simulink model "Robust_design_step_validation_real"  (R2025b)
settings: Solver=ode5  StartTime=0.0  StopTime=20  FixedStep=0.001  RelTol=1e-3
undefined symbols (not defined in the file): degs2rpm, index, K_vec, National_Instruments, Nu, Nx, PCI, rdp, rpm2rads, sens, u_bar_max
libraries: sldrtlib x3
settings Model: SimulationMode=external  ExtModeTrigDuration=20001  Creator=fasoloandr  LastModifiedBy=Enrico
settings DataIOCC: ReturnWorkspaceOutputs=off
settings HardwareCC: ProdBitPerLong=64.0  ProdHWDeviceType=Intel->x86-64 (Linux 64)
settings RTWCC: SystemTargetFile=sldrt.tlc  TemplateMakefile=sldrt.tmf  RTWCompilerOptimization=on  Description=Simulink Desktop Real-Time
settings CodeAppCC: MaxIdLength=95.0
settings SimulinkDesktopRealTimeCC: ExtModeTransport=0.0  ExtModeStaticAllocSize=1000000.0  TargetLibSuffix=_sldrt.a  TargetPreCompLibLocation=D:\Programmi (D)\MATLAB\R2025b\toolbox\sldrt\lib\win64  MultiwordLength=2048.0  DynamicStringBufferSize=256.0  ParMdlRefBuildCompliant=on  PreserveMATLABNamespacesInGeneratedCode=on  SubcomponentCodeInterfacePackaging=Reusable function

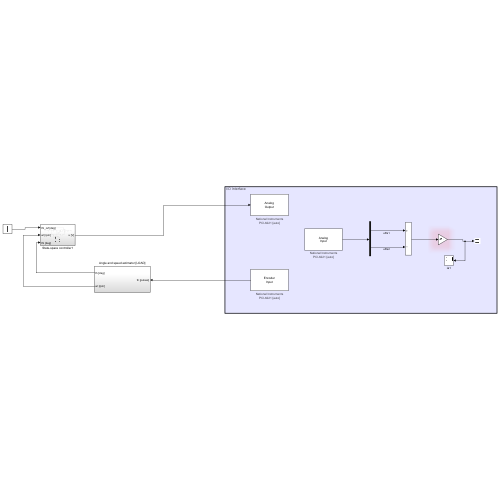
[thumbnail: Simulink's stored preview of the top-level diagram]
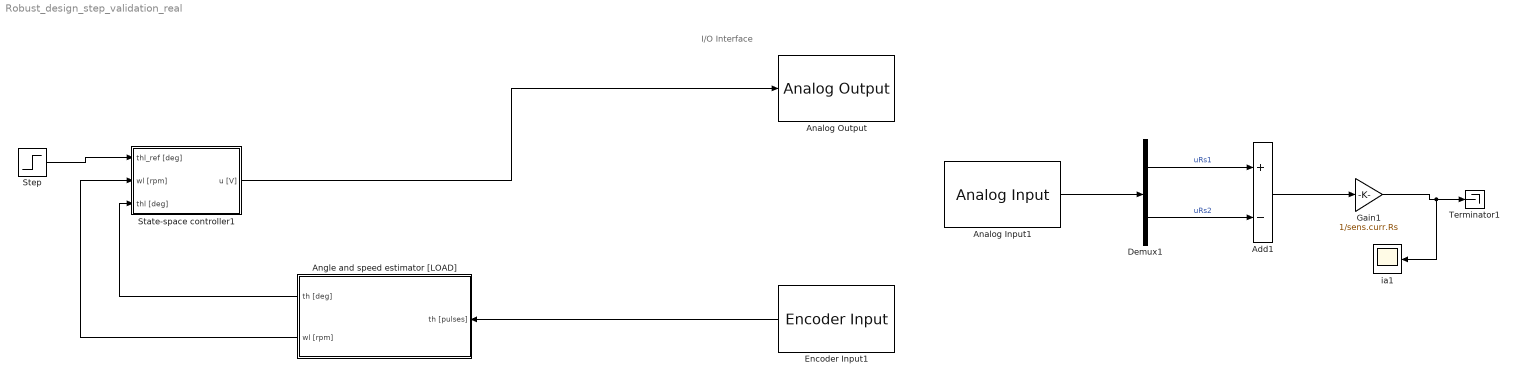
== system Robust_design_step_validation_real ==
  note: I/O Interface
  Add1 : Sum  Inputs=+-
  Analog Input1 : sldrtlib/Analog Input  SampleTime=-1  MaxMissedTicks=10  ShowMissedTicks=off  YieldWhenWaiting=off  DrvName=National_Instruments/PCI-6221  DrvAddress=4294967295  DrvOptions=[0 0 0 2 0]  Channels=[1,2]  RangeMode=1  VoltRange=1  DataType=1
      settings: AttributesFormatString=National Instruments\nPCI-6221 [auto]
  Analog Output : sldrtlib/Analog Output  SampleTime=-1  MaxMissedTicks=10  ShowMissedTicks=off  YieldWhenWaiting=off  DrvName=National_Instruments/PCI-6221  DrvAddress=4294967295  DrvOptions=[0 0 0 2 0]  Channels=1  RangeMode=1  VoltRange=1  InitialValue=[0]  FinalValue=[0]
      settings: AttributesFormatString=National Instruments\nPCI-6221 [auto]
  Angle and speed estimator [LOAD] : Subsystem
  Demux1 : Demux  Outputs=2
  Encoder Input1 : sldrtlib/Encoder Input  SampleTime=-1  MaxMissedTicks=10  ShowMissedTicks=off  YieldWhenWaiting=off  DrvName=National_Instruments/PCI-6221  DrvAddress=4294967295  DrvOptions=[0 0 0 2 0]  Channels=1  QuadMode=3  IndexPulse=1  InputFilter=Inf  DataType=1
      settings: AttributesFormatString=National Instruments\nPCI-6221 [auto]
  Gain1 : Gain  Gain=1/sens.curr.Rs
  State-space controller1 : Subsystem
  Step : Step  SampleTime=0
  Terminator1 : Terminator
  ia1 : Scope
      settings: ActiveDisplayYMinimum=-1  ActiveDisplayYMaximum=1  DataLoggingVariableName=ScopeData2
  wires:
  Add1/1 -> Gain1/1
  Demux1/1 -> Add1/1  "uRs1"
  Demux1/2 -> Add1/2  "uRs2"
  Gain1/1 -> ia1/1, Terminator1/1
  Analog Input1/1 -> Demux1/1
  Step/1 -> State-space controller1/1(thl_ref [deg])
  Angle and speed estimator [LOAD]/1(th [deg]) -> State-space controller1/3(thl [deg])
  Encoder Input1/1 -> Angle and speed estimator [LOAD]/1(th [pulses])
  Angle and speed estimator [LOAD]/2(wl [rpm]) -> State-space controller1/2(wl [rpm])
  State-space controller1/1(u [V]) -> Analog Output/1

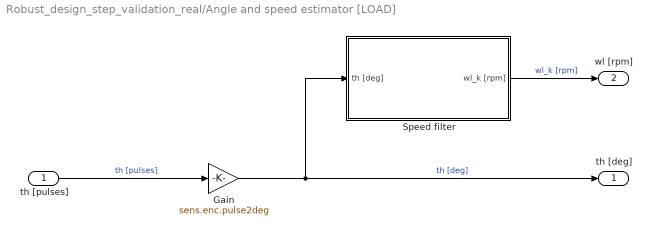
== system Robust_design_step_validation_real/Angle and speed estimator [LOAD] ==
  th [pulses] : Inport
  Gain : Gain  Gain=sens.enc.pulse2deg
  Speed filter : Subsystem
  th [deg] : Outport
  wl [rpm] : Outport  Port=2
  wires:
  Speed filter/1(wl_k [rpm]) -> wl [rpm]/1  "wl_k [rpm]"
  th [pulses]/1 -> Gain/1  "th [pulses]"
  Gain/1 -> Speed filter/1(th [deg]), th [deg]/1  "th [deg]"

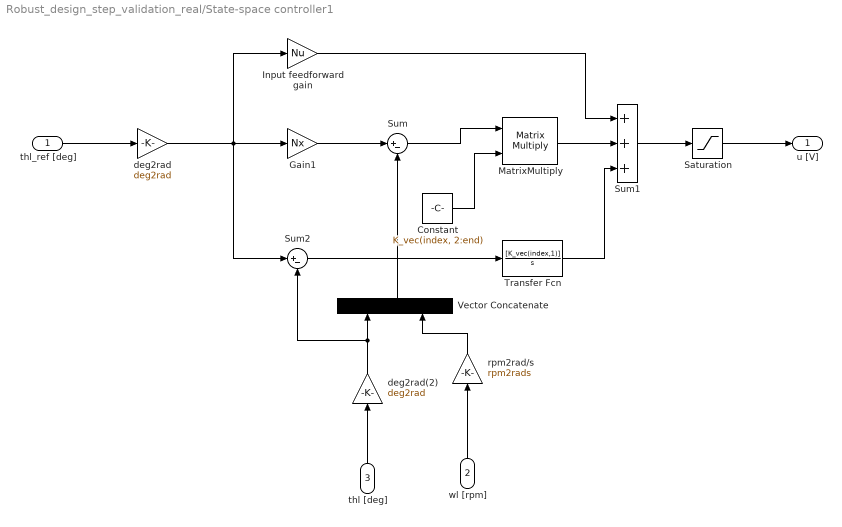
== system Robust_design_step_validation_real/State-space controller1 ==
  thl_ref [deg] : Inport
  wl [rpm] : Inport  Port=2
  thl [deg] : Inport  Port=3
  Constant : Constant  Value=K_vec(index, 2:end)
  Gain1 : Gain  Gain=Nx
  Input feedforward gain : Gain  Gain=Nu
  MatrixMultiply : Product  Multiplication=Matrix(*)
  Saturation : Saturate  UpperLimit=u_bar_max  LowerLimit=-u_bar_max
  Sum : Sum  Inputs=|+-
  Sum1 : Sum  Inputs=+++
  Sum2 : Sum  Inputs=|+-
  Transfer Fcn : TransferFcn  Numerator=[K_vec(index,1)]  Denominator=[1 0]
  Vector Concatenate : Concatenate
  deg2rad : Gain  Gain=deg2rad
  deg2rad(2) : Gain  Gain=deg2rad
  rpm2rad/s : Gain  Gain=rpm2rads
  u [V] : Outport
  wires:
  Gain1/1 -> Sum/1
  Sum1/1 -> Saturation/1
  deg2rad/1 -> Gain1/1, Sum2/1, Input feedforward gain/1
  thl_ref [deg]/1 -> deg2rad/1
  wl [rpm]/1 -> rpm2rad/s/1
  Input feedforward gain/1 -> Sum1/1
  Vector Concatenate/1 -> Sum/2
  Saturation/1 -> u [V]/1
  Sum/1 -> MatrixMultiply/1
  Constant/1 -> MatrixMultiply/2
  MatrixMultiply/1 -> Sum1/2
  Transfer Fcn/1 -> Sum1/3
  Sum2/1 -> Transfer Fcn/1
  thl [deg]/1 -> deg2rad(2)/1
  deg2rad(2)/1 -> Vector Concatenate/1, Sum2/2
  rpm2rad/s/1 -> Vector Concatenate/2

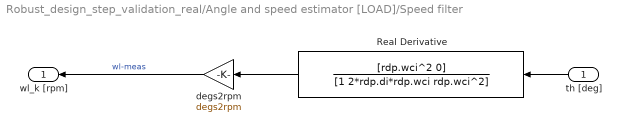
== system Robust_design_step_validation_real/Angle and speed estimator [LOAD]/Speed filter ==
  th [deg] : Inport
  Real Derivative : TransferFcn  Numerator=[rdp.wci^2 0]  Denominator=[1 2*rdp.di*rdp.wci rdp.wci^2]
  degs2rpm : Gain  Gain=degs2rpm
  wl_k [rpm] : Outport
  wires:
  th [deg]/1 -> Real Derivative/1
  degs2rpm/1 -> wl_k [rpm]/1  "wl-meas"
  Real Derivative/1 -> degs2rpm/1
